simulink subsystem "CiEngineCore"  (R2024a)
settings: Solver=VariableStepAuto  StartTime=0.0  StopTime=10.0  RelTol=1e-3
undefined symbols (not defined in the file): EnvCpAir, EnvRair, PlntEngCEng, PlntEngCIEgrArea, PlntEngCISinj, PlntEngCpExh, PlntEngDieselLhv, PlntEngRexh, PlntEngTauCool, PlntEngTCoolInit, PlntEngTCoolMax, PlntEngTCoolStart, ThrAngToC
libraries: autolibfundflw x11, autolibboost x3, autolibcoreeng x1, simulink x1
settings Model: ModifiedByFormat=The MathWorks, Inc.  Creator=The MathWorks, Inc.  LastModifiedBy=The MathWorks, Inc.
settings SolverCC: MaxZcPerStep=1
settings DebuggingCC: UnconnectedInputMsg=warning  UnconnectedOutputMsg=warning  UnconnectedLineMsg=warning
settings ModelReferenceCC: EnableRefExpFcnMdlSchedulingChecks=on
settings RTWCC: GPUComputeCapability=3.5  DLArmComputeVersion=19.05

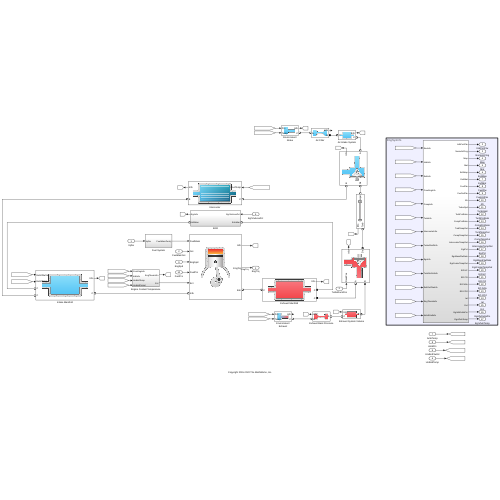
[thumbnail: Simulink's stored preview of the top-level diagram]
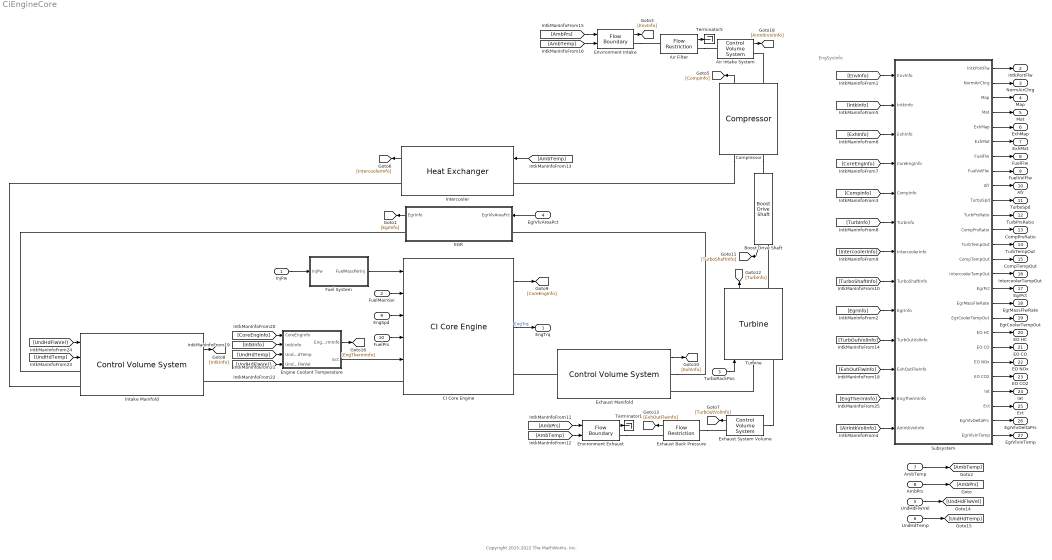
== system CiEngineCore ==
  note: EngSysInfo
  note: Copyright 2015-2022 The MathWorks, Inc.
  InjPw : Inport
  FuelMainSoi : Inport  Port=2
  TurboRackPos : Inport  Port=3
  EgrVlvAreaPct : Inport  Port=4
  UndHdFlwVel : Inport  Port=5
  UndHdTemp : Inport  Port=6
  AmbTemp : Inport  Port=7
  AmbPrs : Inport  Port=8
  EngSpd : Inport  Port=9
  FuelPrs : Inport  Port=10
  Air Filter : autolibfundflw/Flow Restriction  AreaPopup=Constant  ImageTypePopup=Cold  gamma=EnvCpAir/(EnvCpAir-EnvRair)  R=EnvRair  Plim=0.99  Aorf_cnst=PlntEngAFArea  Cd_cnst=1  Cd_ext=1  Dthr=50  ThrCd=[0.001; 0.735]  ThrAngBpts=[0; 90]
  Air Intake System : autolibfundflw/Control Volume System  NumInletPorts=1  NumOutletPorts=1  HeatTransferModelPopup=Constant  ImageTypePopup=Cold  Vch=PlntEngCIAirIntakeVol  Pinit=101325  Tinit=298  R=EnvRair  cp=EnvCpAir  q_he=0  ext_tbl=[40 160 740 2000]  ext_bpts=linspace(0,180,4)  Aext_conv=0.125  m_wall=7  cp_wall=900  Tmass=293.15  Dext_cond=0.004  Aext_cond=0.003  kext=25  Dint_cond=0.004  Aint_cond=0.003  kint=25  int_tbl=[40 160 740 2000]  int_bpts=linspace(0.0020,0.1100,4)  Aint_conv=0.125
  Boost Drive Shaft : autolibboost/Boost Drive Shaft  ShaftConfigPopup=Turbocharger  AddTrqTypePopup=No external torque  J_shaft=PlntEngCITurboInertia  w_0=0.0001  w_min=0.0001  w_max=1e6  eta_mech=1
  CI Core Engine : autolibcoreeng/CI Core Engine  TrqOptionPopup=Torque Structure  NCyl=PlntEngCINCyl  Tstd=EnvAirTemp  Cps=PlntEngCICps  Vd=PlntEngCIVd  Rair=EnvRair  Pstd=EnvAbsPrs  f_nv=PlntEngCINv  f_nv_prs_bpt=PlntEngCINvPrsBpt  f_nv_n_bpt=PlntEngCINvNBpt  f_tq_nf=PlntEngTqNf  f_tq_nf_f_bpt=PlntEngTqNfFBpt  f_tq_nf_n_bpt=PlntEngTqNfNBpt  f_tqs_f_bpt=PlntEngCIGIMepFuelBpt  f_tqs_n_bpt=PlntEngCIGIMepSpdBpt  f_tqs_mainsoi=PlntEngTqsMainSoi  f_tqs_map=PlntEngTqsMap  f_tqs_emap=PlntEngTqsEMap  f_tqs_mat=PlntEngTqsMat  f_tqs_o2pct=PlntEngTqsO2Pct  f_tqs_fuelpress=PlntEngTqsFuelPres  f_tqs_imepg=PlntEngCIGIMepMap  f_tqs_fmep=PlntEngTqsFMep  f_tqs_pmep=PlntEngTqsPMEP  f_tqs_fric_temp_mod=PlntEngTqsFrTmpMod  f_tqs_fric_temp_bpt=PlntEngTqsFrTmpBpt  f_tqs_mainsoi_eff=PlntEngTqsMainSoiEff  f_tqs_mainsoi_delta_bpt=PlntEngTqsMainSoiDeltaBpt  f_tqs_map_eff=PlntEngTqsMapEff  f_tqs_map_ratio_bpt=PlntEngTqsMapRatioBpt  f_tqs_lambda_bpt=PlntEngTqsLambdaBpt  f_tqs_mat_eff=PlntEngTqsMatEff  f_tqs_mat_delta_bpt=PlntEngTqsMatDeltaBpt  f_tqs_o2pct_eff=PlntEngTqsO2PctEff  f_tqs_o2pct_delta_bpt=PlntEngTqsO2PctDeltaBpt  f_tqs_fuelpress_eff=PlntEngTqsFuelPrsEff  f_tqs_fuelpress_delta_bpt=PlntEngTqsFuelPrsDeltaBpt  f_tqs_f_inj_type=PlntEngTqsInjType  f_tqs_imep_post_corr=PlntEngTqsImepPostCorr  f_tqs_f_post_sum_bpt=PlntEngTqsPostSumBpt  f_tqs_soi_post_cent_bpt=PlntEngTqsSoiPostCenBpt  f_tqs_f_burned_soi_limit=PlntEngTqsBurnedSoiLim  f_t_exh=PlntEngCITexh  f_t_exh_f_bpt=PlntEngCITexhFBpt  f_t_exh_n_bpt=PlntEngCITexhNBpt  f_tqs_exht=PlntEngTqsExhT  f_tqs_exht_mainsoi_eff=PlntEngTqsExhTMainSoiEff  f_tqs_exht_map_eff=PlntEngTqsExhTMapEff  f_tqs_exht_mat_eff=PlntEngTqsExhTMatEff  f_tqs_exht_o2pct_eff=PlntEngTqsExhTO2PctEff  f_tqs_exht_fuelpress_eff=PlntEngTqsExhTFuelPrsEff  f_tqs_exht_post_inj_wall_htc=PlntEngTqsExhTPstInjWHtc  CO2EmissionsCheckbox=on  COEmissionsCheckbox=on  NOxEmissionsCheckbox=on  HCEmissionsCheckbox=on  PMEmissionsCheckbox=off  f_CO2_frac=PlntEngCICorefCO2  f_CO_frac=PlntEngCICorefCO  f_HC_frac=PlntEngCICorefHC  f_NOx_frac=PlntEngCICorefNOx  f_PM_frac=[0 0 0 0 0 0 0 0 0 0 0 0 0 0 0;0 0 0 0 0 0 0 0 0 0 0 0 0 0 0;0 0 0 0 0 0 0 0 0 0 0 0 0 0 0;0 0 0 0 0 0 0 0 0 0 0 0 0 0 0;0 0 0 0 0 0 0 0 0 0 0 0 0 0 0;0 0 0 0 0 0 0 0 0 0 0 0 0 0 0;0 0 0 0 0 0 0 0 0 0 0 0 0 0 0;0 0 0 0 0 0 0 0 0 0 0 0 0 0 0;0 0 0 0 0 0 0 0 0 0 0 0 0 0 0;0 0 0 0 0 0 0 0 0 0 0 0 0 0 0;0 0 0 0 0 0 0 0 0 0 0 0 0 0 0;0 0 0 0 0 0 0 0 0 0 0 0 0 0 0;0 0 0 0 0 0 0 0 0 0 0 0 0 0 0;0 0 0 0 0 0 0 0 0 0 0 0 0 0 0;0 0 0 0 0 0 0 0 0 0 0 0 0 0 0;0 0 0 0 0 0 0 0 0 0 0 0 0 0 0]  f_exhfrac_n_bpt=PlntEngCIExhFracNBpt  f_exhfrac_trq_bpt=PlntEngCIExhFracTqBpt  cp_exh=PlntEngCpExh  afr_stoich=PlntEngAfrStoich  fuel_lhv=PlntEngDieselLhv  fuel_sg=0.832
  Compressor : autolibboost/Compressor  mdot_corr_tbl=PlntEngCICompMassFlwRate  eta_comp_tbl=PlntEngCICompEff  w_corr_bpts1=PlntEngCICompSpdBreakPoints  Pr_bpts2=PlntEngCmpPrBpt  T_ref=PlntEngCmpRefT  P_ref=PlntEngCmpRefP  R=EnvRair  cp=EnvCpAir  CalCmprsData={'', '', 'MassFlwRate', 'Eff'}
  EGR : Subsystem
  Engine Coolant Temperature : Subsystem
  Environment Exhaust : autolibfundflw/Flow Boundary  PrsTempSrcPopup=External input  ImageTypePopup=Hot  Pcnst=101325  Tcnst=298.15  cp=EnvCpAir
  Environment Intake : autolibfundflw/Flow Boundary  PrsTempSrcPopup=External input  ImageTypePopup=Cold  Pcnst=101325  Tcnst=298.15  cp=EnvCpAir
  Exhaust Back Pressure : autolibfundflw/Flow Restriction  AreaPopup=Constant  ImageTypePopup=Hot  gamma=PlntEngCpExh/(PlntEngCpExh-PlntEngRexh)  R=PlntEngRexh  Plim=0.99  Aorf_cnst=PlntEngCIExhSysArea  Cd_cnst=1  Cd_ext=1  Dthr=50  ThrCd=[0.001; 0.735]  ThrAngBpts=[0; 90]
  Exhaust Manifold : autolibfundflw/Control Volume System  NumInletPorts=1  NumOutletPorts=2  HeatTransferModelPopup=Constant  ImageTypePopup=Hot  Vch=PlntEngCIVexh  Pinit=101325  Tinit=298  R=PlntEngRexh  cp=PlntEngCpExh  q_he=0  ext_tbl=[40 160 740 2000]  ext_bpts=linspace(0,180,4)  Aext_conv=0.125  m_wall=7  cp_wall=900  Tmass=293.15  Dext_cond=0.004  Aext_cond=0.003  kext=25  Dint_cond=0.004  Aint_cond=0.003  kint=25  int_tbl=[40 160 740 2000]  int_bpts=linspace(0.0020,0.1100,4)  Aint_conv=0.125
  Exhaust System Volume : autolibfundflw/Control Volume System  NumInletPorts=1  NumOutletPorts=1  HeatTransferModelPopup=Constant  ImageTypePopup=Hot  Vch=PlntEngCIExhSysVol  Pinit=101325  Tinit=298  R=PlntEngRexh  cp=PlntEngCpExh  q_he=0  ext_tbl=[40 160 740 2000]  ext_bpts=linspace(0,180,4)  Aext_conv=0.125  m_wall=7  cp_wall=900  Tmass=293.15  Dext_cond=0.004  Aext_cond=0.003  kext=25  Dint_cond=0.004  Aint_cond=0.003  kint=25  int_tbl=[40 160 740 2000]  int_bpts=linspace(0.0020,0.1100,4)  Aint_conv=0.125
  Fuel System : Subsystem
  Intake Manifold : autolibfundflw/Control Volume System  NumInletPorts=2  NumOutletPorts=1  HeatTransferModelPopup=External wall convection  ImageTypePopup=Cold  Vch=PlntEngCIVint  Pinit=101325  Tinit=298  R=EnvRair  cp=EnvCpAir  q_he=0  ext_tbl=[40 160 740 2000]  ext_bpts=linspace(0,180,4)  Aext_conv=0.125  m_wall=7  cp_wall=900  Tmass=293.15  Dext_cond=0.004  Aext_cond=0.003  kext=25  Dint_cond=0.004  Aint_cond=0.003  kint=25  int_tbl=[40 160 740 2000]  int_bpts=linspace(0.0020,0.1100,4)  Aint_conv=0.125
  Intercooler : autolibfundflw/Heat Exchanger  EffctModelPopup=Constant  CoolTempInputPopup=External input  ImageTypePopup=Intercooler  ep_cnst=PlntEngCIIcEffectiveness  T_cool_cnst=PlntEngCoolTemp  cp=EnvCpAir
  Subsystem : Subsystem
  Terminator1 : Terminator
  Terminator5 : Terminator
  Turbine : autolibboost/Turbine  TurbTypePopup=Variable geometry  WgIncludeCheckbox=off  mdot_corrfx_tbl=TurbMassFlwRate  mdot_corrvr_tbl=PlntEngCITurbMassFlwRate  eta_turbfx_tbl=TurbEff  eta_turbvr_tbl=PlntEngCITurbEff  w_corrfx_bpts1=TurbSpdBreakPoints  w_corrvr_bpts2=PlntEngCITurbSpdBreakPoints  Pr_fx_bpts2=TurbPrsRatioBreakPoints  Pr_vr_bpts2=PlntEngCITurbPrsRatioBreakPoints  L_rack_bpts3=PlntEngCITurbRackBreakPoints  T_ref=PlntEngTrbRefT  P_ref=PlntEngTrbRefP  mdot_thresh=1e-6  A_wgopen=WgArea  Plim_wg=.99  R=PlntEngRexh  cp=PlntEngCpExh  CalFixedMapsData={'', '', 'FixedTurbine'}  CalVgtMapsData={'', '', 'Vgt-Point-by-Point'}
  EngTrq : Outport  VectorParamsAs1DForOutWhenUnconnected=off
  IntkPortFlw : Outport  Port=2  VectorParamsAs1DForOutWhenUnconnected=off
  NormAirChrg : Outport  Port=3  VectorParamsAs1DForOutWhenUnconnected=off
  Map : Outport  Port=4  VectorParamsAs1DForOutWhenUnconnected=off
  Mat : Outport  Port=5  VectorParamsAs1DForOutWhenUnconnected=off
  ExhMap : Outport  Port=6  VectorParamsAs1DForOutWhenUnconnected=off
  ExhMat : Outport  Port=7  VectorParamsAs1DForOutWhenUnconnected=off
  FuelFlw : Outport  Port=8  VectorParamsAs1DForOutWhenUnconnected=off
  FuelVolFlw : Outport  Port=9  VectorParamsAs1DForOutWhenUnconnected=off
  Afr : Outport  Port=10  VectorParamsAs1DForOutWhenUnconnected=off
  TurboSpd : Outport  Port=11  VectorParamsAs1DForOutWhenUnconnected=off
  TurbPrsRatio : Outport  Port=12  VectorParamsAs1DForOutWhenUnconnected=off
  CompPrsRatio : Outport  Port=13  VectorParamsAs1DForOutWhenUnconnected=off
  TurbTempOut : Outport  Port=14  VectorParamsAs1DForOutWhenUnconnected=off
  CompTempOut : Outport  Port=15  VectorParamsAs1DForOutWhenUnconnected=off
  IntercoolerTempOut : Outport  Port=16  VectorParamsAs1DForOutWhenUnconnected=off
  EgrPct : Outport  Port=17  VectorParamsAs1DForOutWhenUnconnected=off
  EgrMassFlwRate : Outport  Port=18  VectorParamsAs1DForOutWhenUnconnected=off
  EgrCoolerTempOut : Outport  Port=19  VectorParamsAs1DForOutWhenUnconnected=off
  EO HC : Outport  Port=20  VectorParamsAs1DForOutWhenUnconnected=off
  EO CO : Outport  Port=21  VectorParamsAs1DForOutWhenUnconnected=off
  EO NOx : Outport  Port=22  VectorParamsAs1DForOutWhenUnconnected=off
  EO CO2 : Outport  Port=23  VectorParamsAs1DForOutWhenUnconnected=off
  Iat : Outport  Port=24  VectorParamsAs1DForOutWhenUnconnected=off
  Ect : Outport  Port=25  VectorParamsAs1DForOutWhenUnconnected=off
  EgrVlvDeltaPrs : Outport  Port=26  VectorParamsAs1DForOutWhenUnconnected=off
  EgrVlvInTemp : Outport  Port=27  VectorParamsAs1DForOutWhenUnconnected=off
  wires:
  Subsystem/16(EgrPct) -> EgrPct/1
  Environment Exhaust/1 -> Terminator1/1
  InjPw/1 -> Fuel System/1(InjPw)
  TurboRackPos/1 -> Turbine/1
  Engine Coolant Temperature/2(Ect) -> CI Core Engine/5
  Engine Coolant Temperature/1(EngThermInfo) -> [EngThermInfo]
  UndHdTemp/1 -> [UndHdTemp]
  [UndHdFlwVel] -> Intake Manifold/1
  [IntkInfo] -> Engine Coolant Temperature/2(IntkInfo)
  Subsystem/13(TurbTempOut) -> TurbTempOut/1
  Turbine/1 -> [TurbInfo]
  UndHdFlwVel/1 -> [UndHdFlwVel]
  Subsystem/19(EO HC) -> EO HC/1
  [CoreEngInfo] -> Engine Coolant Temperature/1(CoreEngInfo)
  Subsystem/18(EgrCoolerTempOut) -> EgrCoolerTempOut/1
  Subsystem/24(Ect) -> Ect/1
  [TurboShaftInfo] -> Subsystem/8(TurboShaftInfo)
  Subsystem/6(ExhMat) -> ExhMat/1
  Subsystem/4(Mat) -> Mat/1
  [UndHdTemp] -> Engine Coolant Temperature/3(UndHdTemp)
  Fuel System/1(FuelMassPerInj) -> CI Core Engine/1
  [UndHdFlwVel] -> Engine Coolant Temperature/4(UndHdFlwVel)
  [EgrInfo] -> Subsystem/9(EgrInfo)
  [ExhOutFlwInfo] -> Subsystem/11(ExhOutFlwInfo)
  Subsystem/20(EO CO) -> EO CO/1
  [AmbTemp] -> Environment Intake/2
  Subsystem/11(TurbPrsRatio) -> TurbPrsRatio/1
  FuelMainSoi/1 -> CI Core Engine/2
  [TurbOutVolInfo] -> Subsystem/10(TurbOutVolInfo)
  Subsystem/15(IntercoolerTempOut) -> IntercoolerTempOut/1
  Subsystem/17(EgrMassFlwRate) -> EgrMassFlwRate/1
  Subsystem/2(NormAirChrg) -> NormAirChrg/1
  [CoreEngInfo] -> Subsystem/4(CoreEngInfo)
  [AmbPrs] -> Environment Intake/1
  Subsystem/5(ExhMap) -> ExhMap/1
  Subsystem/9(Afr) -> Afr/1
  AmbTemp/1 -> [AmbTemp]
  Environment Intake/1 -> [EnvInfo]
  [TurbInfo] -> Subsystem/6(TurbInfo)
  Subsystem/1(IntkPortFlw) -> IntkPortFlw/1
  CI Core Engine/1 -> [CoreEngInfo]
  [ExhInfo] -> Subsystem/3(ExhInfo)
  [EnvInfo] -> Subsystem/1(EnvInfo)
  [IntkInfo] -> Subsystem/2(IntkInfo)
  [AmbPrs] -> Environment Exhaust/1
  Exhaust Manifold/1 -> [ExhInfo]
  AmbPrs/1 -> [AmbPrs]
  [CompInfo] -> Subsystem/5(CompInfo)
  Subsystem/21(EO NOx) -> EO NOx/1
  Subsystem/3(Map) -> Map/1
  [AmbTemp] -> Intercooler/1
  EgrVlvAreaPct/1 -> EGR/1(EgrVlvAreaPct)
  EngSpd/1 -> CI Core Engine/3
  Compressor/1 -> [CompInfo]
  Air Filter/1 -> Terminator5/1
  Exhaust Back Pressure/1 -> [ExhOutFlwInfo]
  [EngThermInfo] -> Subsystem/12(EngThermInfo)
  Air Intake System/1 -> [AirIntkVolInfo]
  Intake Manifold/1 -> [IntkInfo]
  Subsystem/8(FuelVolFlw) -> FuelVolFlw/1
  Exhaust System Volume/1 -> [TurbOutVolInfo]
  Subsystem/14(CompTempOut) -> CompTempOut/1
  Subsystem/22(EO CO2) -> EO CO2/1
  EGR/1(EgrInfo) -> [EgrInfo]
  [AmbTemp] -> Environment Exhaust/2
  Subsystem/10(TurboSpd) -> TurboSpd/1
  FuelPrs/1 -> CI Core Engine/4
  Subsystem/12(CompPrsRatio) -> CompPrsRatio/1
  Subsystem/23(Iat) -> Iat/1
  CI Core Engine/2 -> EngTrq/1  "EngTrq"
  [IntercoolerInfo] -> Subsystem/7(IntercoolerInfo)
  [UndHdTemp] -> Intake Manifold/2
  [AirIntkVolInfo] -> Subsystem/13(AirIntkVolInfo)
  Subsystem/25(EgrVlvDeltaPrs) -> EgrVlvDeltaPrs/1
  Intercooler/1 -> [IntercoolerInfo]
  Subsystem/7(FuelFlw) -> FuelFlw/1
  Subsystem/26(EgrVlvInTemp) -> EgrVlvInTemp/1
  Boost Drive Shaft/1 -> [TurboShaftInfo]
  connections:
  Exhaust System Volume/LConn1 -- Turbine/LConn2
  Turbine/LConn1 -- Exhaust Manifold/RConn2
  Exhaust Manifold/LConn1 -- CI Core Engine/RConn1
  Exhaust Back Pressure/LConn1 -- Exhaust System Volume/RConn1
  Intake Manifold/LConn1 -- EGR/RConn1
  Environment Intake/RConn1 -- Air Filter/LConn1
  Compressor/LConn1 -- Intercooler/LConn1
  Exhaust Manifold/RConn1 -- EGR/LConn1
  Intercooler/RConn1 -- Intake Manifold/LConn2
  Compressor/RConn1 -- Air Intake System/RConn1
  Environment Exhaust/RConn1 -- Exhaust Back Pressure/RConn1
  CI Core Engine/LConn1 -- Intake Manifold/RConn1
  Compressor/LConn2 -- Boost Drive Shaft/LConn1
  Air Filter/RConn1 -- Air Intake System/LConn1
  Turbine/RConn1 -- Boost Drive Shaft/RConn1

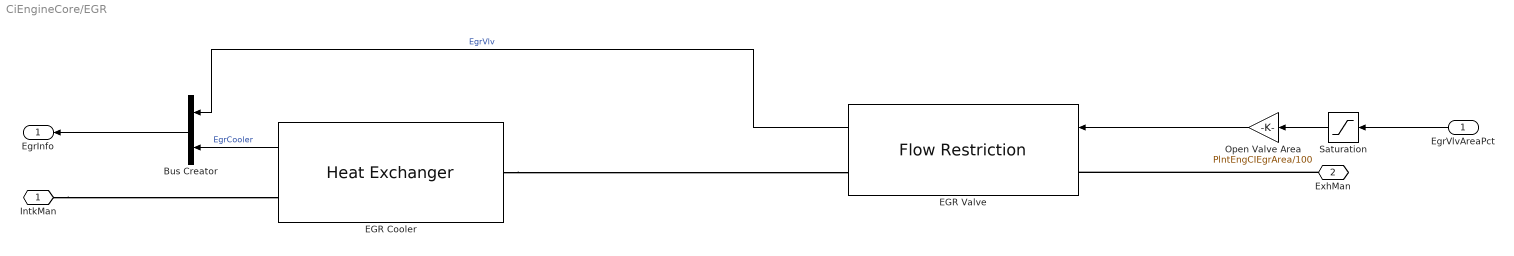
== system CiEngineCore/EGR ==
  EgrVlvAreaPct : Inport
  Bus Creator : BusCreator  Inputs=2
  EGR Cooler : autolibfundflw/Heat Exchanger  EffctModelPopup=Constant  CoolTempInputPopup=Constant  ImageTypePopup=EGR cooler hot to cold  ep_cnst=PlntEngEgrEff  T_cool_cnst=PlntEngREgrCoolT  cp=PlntEngCpExh
  EGR Valve : autolibfundflw/Flow Restriction  AreaPopup=External input  ImageTypePopup=Hot  gamma=PlntEngCpExh / (PlntEngCpExh - PlntEngRexh)  R=EnvRair  Plim=0.99  Aorf_cnst=.1  Cd_cnst=1  Cd_ext=1  Dthr=ThrDiam  ThrCd=ThrAngToC(:,2)  ThrAngBpts=ThrAngToC(:,1)
  Open Valve Area : Gain  Gain=PlntEngCIEgrArea/100
  Saturation : Saturate  UpperLimit=100  LowerLimit=0
  IntkMan : PMIOPort  Side=Right
  ExhMan : PMIOPort  Port=2  Side=Left
  EgrInfo : Outport  VectorParamsAs1DForOutWhenUnconnected=off
  wires:
  EgrVlvAreaPct/1 -> Saturation/1
  Open Valve Area/1 -> EGR Valve/1
  Saturation/1 -> Open Valve Area/1
  Bus Creator/1 -> EgrInfo/1
  EGR Cooler/1 -> Bus Creator/2  "EgrCooler"
  EGR Valve/1 -> Bus Creator/1  "EgrVlv"
  connections:
  EGR Cooler/LConn1 -- EGR Valve/RConn1
  IntkMan/RConn1 -- EGR Cooler/RConn1
  ExhMan/RConn1 -- EGR Valve/LConn1

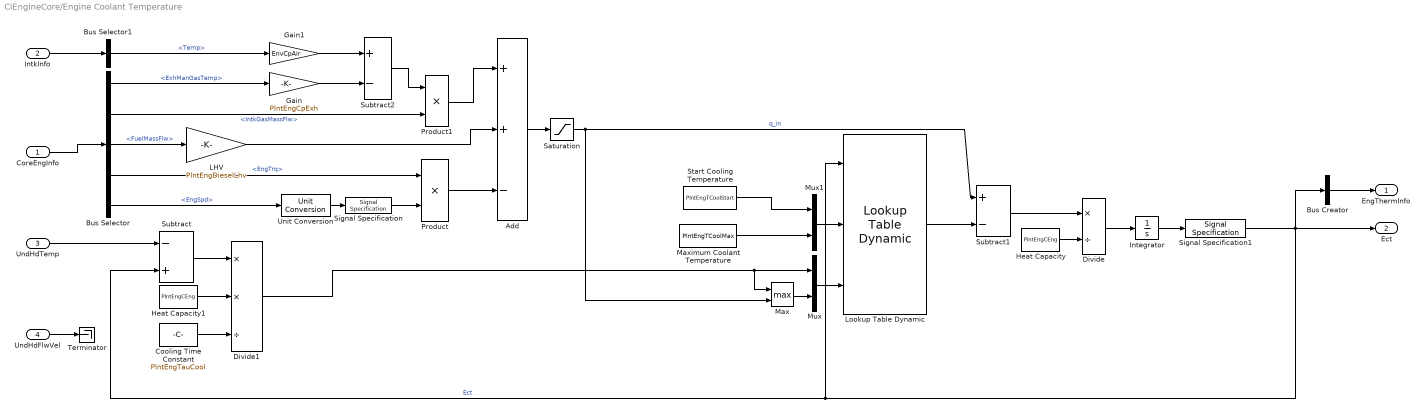
== system CiEngineCore/Engine Coolant Temperature ==
  CoreEngInfo : Inport
  IntkInfo : Inport  Port=2
  UndHdTemp : Inport  Port=3
  UndHdFlwVel : Inport  Port=4
  Add : Sum  Inputs=++-
  Bus Creator : BusCreator  Inputs=1
  Bus Selector : BusSelector  OutputSignals=ExhManGasTemp,IntkGasMassFlw,FuelMassFlw,EngTrq,EngSpd
  Bus Selector1 : BusSelector  OutputSignals=Vol.Temp
  Cooling Time Constant : Constant  Value=PlntEngTauCool
  Divide : Product  Inputs=*/
  Divide1 : Product  Inputs=**/
  Gain : Gain  Gain=PlntEngCpExh
  Gain1 : Gain  Gain=EnvCpAir
  Heat Capacity : Constant  Value=PlntEngCEng
  Heat Capacity1 : Constant  Value=PlntEngCEng
  Integrator : Integrator  InitialCondition=PlntEngTCoolInit  LimitOutput=on  UpperSaturationLimit=PlntEngTCoolMax  LowerSaturationLimit=0  ZeroCross=off
  LHV : Gain  Gain=PlntEngDieselLhv
  Lookup Table Dynamic : simulink/Lookup Tables/Lookup Table Dynamic  LookUpMeth=Interpolation-Use End Values  OutDataType=fixdt('double')  OutScaling=[]  OutputDataTypeScalingMode=Specify via dialog  OutDataTypeStr=double  DoSatur=off
  Max : MinMax  Function=max  Inputs=2  ZeroCross=off
  Maximum Coolant Temperature : Constant  Value=PlntEngTCoolMax
  Mux : Mux  Inputs=2
  Mux1 : Mux  Inputs=2
  Product : Product
  Product1 : Product
  Saturation : Saturate  UpperLimit=Inf  LowerLimit=0
  Signal Specification : SignalSpecification  Unit=rad/s
  Signal Specification1 : SignalSpecification  Unit=K
  Start Cooling Temperature : Constant  Value=PlntEngTCoolStart
  Subtract : Sum  Inputs=-+
  Subtract1 : Sum  Inputs=+-
  Subtract2 : Sum  Inputs=+-
  Terminator : Terminator
  Unit Conversion : UnitConversion
  EngThermInfo : Outport  Unit=K  VectorParamsAs1DForOutWhenUnconnected=off
  Ect : Outport  Port=2  Unit=K  VectorParamsAs1DForOutWhenUnconnected=off
  wires:
  UndHdTemp/1 -> Subtract/1
  Heat Capacity/1 -> Divide/2
  Unit Conversion/1 -> Signal Specification/1
  Maximum Coolant Temperature/1 -> Mux1/2
  Signal Specification1/1 -> Subtract/2, Lookup Table Dynamic/1, Bus Creator/1, Ect/1  "Ect"
  UndHdFlwVel/1 -> Terminator/1
  Gain/1 -> Subtract2/2
  Bus Selector/4 -> Product/1  "<EngTrq>"
  Mux1/1 -> Lookup Table Dynamic/2
  Divide1/1 -> Max/1, Mux/1
  Heat Capacity1/1 -> Divide1/2
  Mux/1 -> Lookup Table Dynamic/3
  Start Cooling Temperature/1 -> Mux1/1
  Subtract/1 -> Divide1/1
  Saturation/1 -> Max/2, Subtract1/1  "q_in"
  Signal Specification/1 -> Product/2
  LHV/1 -> Add/2
  Product/1 -> Add/3
  Bus Selector/5 -> Unit Conversion/1  "<EngSpd>"
  Cooling Time Constant/1 -> Divide1/3
  CoreEngInfo/1 -> Bus Selector/1
  Bus Selector/3 -> LHV/1  "<FuelMassFlw>"
  Bus Selector/1 -> Gain/1  "<ExhManGasTemp>"
  Gain1/1 -> Subtract2/1
  Bus Selector1/1 -> Gain1/1  "<Temp>"
  Divide/1 -> Integrator/1
  Subtract1/1 -> Divide/1
  Lookup Table Dynamic/1 -> Subtract1/2
  Max/1 -> Mux/2
  Bus Creator/1 -> EngThermInfo/1
  IntkInfo/1 -> Bus Selector1/1
  Integrator/1 -> Signal Specification1/1
  Subtract2/1 -> Product1/1
  Bus Selector/2 -> Product1/2  "<IntkGasMassFlw>"
  Product1/1 -> Add/1
  Add/1 -> Saturation/1

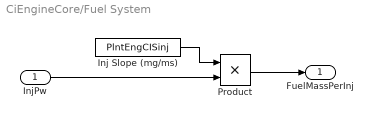
== system CiEngineCore/Fuel System ==
  InjPw : Inport
  Inj Slope (mg/ms) : Constant  Value=PlntEngCISinj
  Product : Product
  FuelMassPerInj : Outport  VectorParamsAs1DForOutWhenUnconnected=off
  wires:
  InjPw/1 -> Product/2
  Inj Slope (mg/ms)/1 -> Product/1
  Product/1 -> FuelMassPerInj/1

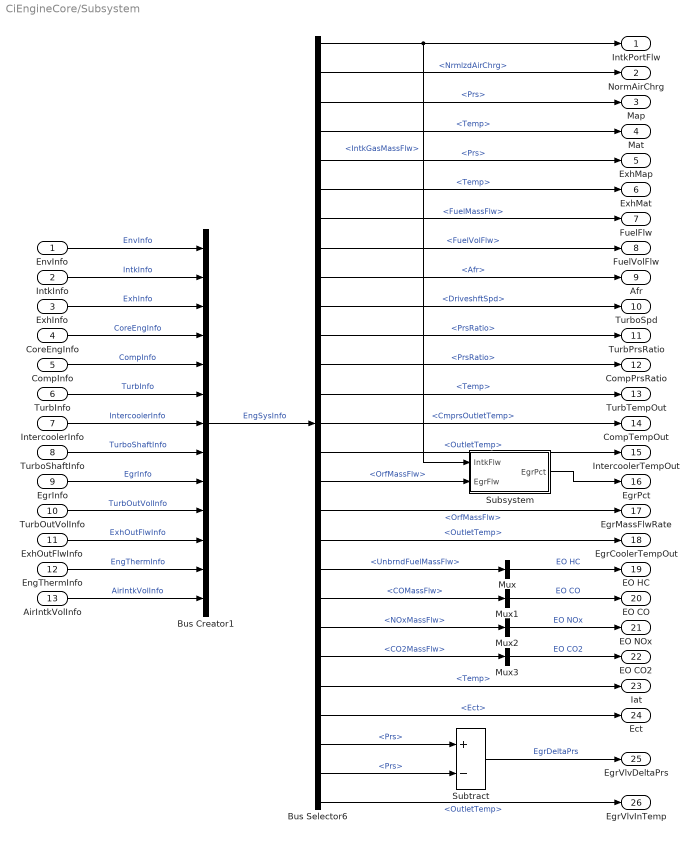
== system CiEngineCore/Subsystem ==
  EnvInfo : Inport
  IntkInfo : Inport  Port=2
  ExhInfo : Inport  Port=3
  CoreEngInfo : Inport  Port=4
  CompInfo : Inport  Port=5
  TurbInfo : Inport  Port=6
  IntercoolerInfo : Inport  Port=7
  TurboShaftInfo : Inport  Port=8
  EgrInfo : Inport  Port=9
  TurbOutVolInfo : Inport  Port=10
  ExhOutFlwInfo : Inport  Port=11
  EngThermInfo : Inport  Port=12
  AirIntkVolInfo : Inport  Port=13
  Bus Creator1 : BusCreator  Inputs=13
  Bus Selector6 : BusSelector  OutputSignals=CoreEngInfo.IntkGasMassFlw,CoreEngInfo.NrmlzdAirChrg,IntkInfo.Vol.Prs,IntkInfo.Vol.Temp,ExhInfo.Vol.Prs,ExhInfo.Vol.Temp,CoreEngInfo.FuelMassFlw,CoreEngInfo.FuelVolFlw,CoreEngInfo.Afr,TurboShaftInfo.DriveshftSpd,TurbInfo.PrsRatio,CompInfo.PrsRatio,TurbOutVolInfo.Vol.Temp,CompInfo.CmprsOutletTemp,IntercoolerInfo.OutletTemp,EgrInfo.EgrVlv.Flw.OrfMassFlw,EgrInfo.EgrVlv.Flw.OrfMassFlw,EgrInfo.EgrCooler.OutletTemp,ExhOutFlwInfo.Flw.Species.UnbrndFuelMassFlw,ExhOutFlwInfo.Flw.Species.COMassFlw,ExhOutFlwInfo.Flw.Species.NOxMassFlw,ExhOutFlwInfo.Flw.Species.CO2MassFlw,AirIntkVolInfo.Vol.Temp,EngThermInfo.Ect,ExhInfo.Vol.Prs,IntkInfo.Vol.Prs,EgrInfo.EgrCooler.OutletTemp
  Mux{,1..3} (4 alike) : Mux  Inputs=1
  Subsystem : Subsystem
  Subtract : Sum  Inputs=+-
  IntkPortFlw : Outport  VectorParamsAs1DForOutWhenUnconnected=off
  NormAirChrg : Outport  Port=2  Unit=1  VectorParamsAs1DForOutWhenUnconnected=off
  Map : Outport  Port=3  VectorParamsAs1DForOutWhenUnconnected=off
  Mat : Outport  Port=4  VectorParamsAs1DForOutWhenUnconnected=off
  ExhMap : Outport  Port=5  VectorParamsAs1DForOutWhenUnconnected=off
  ExhMat : Outport  Port=6  VectorParamsAs1DForOutWhenUnconnected=off
  FuelFlw : Outport  Port=7  VectorParamsAs1DForOutWhenUnconnected=off
  FuelVolFlw : Outport  Port=8  VectorParamsAs1DForOutWhenUnconnected=off
  Afr : Outport  Port=9  Unit=1  VectorParamsAs1DForOutWhenUnconnected=off
  TurboSpd : Outport  Port=10  VectorParamsAs1DForOutWhenUnconnected=off
  TurbPrsRatio : Outport  Port=11  VectorParamsAs1DForOutWhenUnconnected=off
  CompPrsRatio : Outport  Port=12  VectorParamsAs1DForOutWhenUnconnected=off
  TurbTempOut : Outport  Port=13  VectorParamsAs1DForOutWhenUnconnected=off
  CompTempOut : Outport  Port=14  VectorParamsAs1DForOutWhenUnconnected=off
  IntercoolerTempOut : Outport  Port=15  VectorParamsAs1DForOutWhenUnconnected=off
  EgrPct : Outport  Port=16  Unit=%  VectorParamsAs1DForOutWhenUnconnected=off
  EgrMassFlwRate : Outport  Port=17  VectorParamsAs1DForOutWhenUnconnected=off
  EgrCoolerTempOut : Outport  Port=18  VectorParamsAs1DForOutWhenUnconnected=off
  EO HC : Outport  Port=19  VectorParamsAs1DForOutWhenUnconnected=off
  EO CO : Outport  Port=20  VectorParamsAs1DForOutWhenUnconnected=off
  EO NOx : Outport  Port=21  VectorParamsAs1DForOutWhenUnconnected=off
  EO CO2 : Outport  Port=22  VectorParamsAs1DForOutWhenUnconnected=off
  Iat : Outport  Port=23  VectorParamsAs1DForOutWhenUnconnected=off
  Ect : Outport  Port=24  VectorParamsAs1DForOutWhenUnconnected=off
  EgrVlvDeltaPrs : Outport  Port=25  Unit=Pa  VectorParamsAs1DForOutWhenUnconnected=off
  EgrVlvInTemp : Outport  Port=26  Unit=K  VectorParamsAs1DForOutWhenUnconnected=off
  wires:
  TurbOutVolInfo/1 -> Bus Creator1/10  "TurbOutVolInfo"
  EgrInfo/1 -> Bus Creator1/9  "EgrInfo"
  Bus Selector6/15 -> IntercoolerTempOut/1  "<OutletTemp>"
  Bus Selector6/14 -> CompTempOut/1  "<CmprsOutletTemp>"
  Bus Selector6/13 -> TurbTempOut/1  "<Temp>"
  Bus Selector6/12 -> CompPrsRatio/1  "<PrsRatio>"
  Bus Selector6/11 -> TurbPrsRatio/1  "<PrsRatio>"
  Bus Selector6/2 -> NormAirChrg/1  "<NrmlzdAirChrg>"
  Bus Selector6/9 -> Afr/1  "<Afr>"
  Bus Selector6/7 -> FuelFlw/1  "<FuelMassFlw>"
  Bus Selector6/6 -> ExhMat/1  "<Temp>"
  Bus Selector6/5 -> ExhMap/1  "<Prs>"
  Bus Selector6/4 -> Mat/1  "<Temp>"
  Bus Selector6/3 -> Map/1  "<Prs>"
  Bus Selector6/1 -> Subsystem/1(IntkFlw), IntkPortFlw/1  "<IntkGasMassFlw>"
  TurboShaftInfo/1 -> Bus Creator1/8  "TurboShaftInfo"
  TurbInfo/1 -> Bus Creator1/6  "TurbInfo"
  IntercoolerInfo/1 -> Bus Creator1/7  "IntercoolerInfo"
  Bus Creator1/1 -> Bus Selector6/1  "EngSysInfo"
  EnvInfo/1 -> Bus Creator1/1  "EnvInfo"
  CoreEngInfo/1 -> Bus Creator1/4  "CoreEngInfo"
  ExhInfo/1 -> Bus Creator1/3  "ExhInfo"
  IntkInfo/1 -> Bus Creator1/2  "IntkInfo"
  CompInfo/1 -> Bus Creator1/5  "CompInfo"
  Bus Selector6/18 -> EgrCoolerTempOut/1  "<OutletTemp>"
  ExhOutFlwInfo/1 -> Bus Creator1/11  "ExhOutFlwInfo"
  Bus Selector6/19 -> Mux/1  "<UnbrndFuelMassFlw>"
  Bus Selector6/20 -> Mux1/1  "<COMassFlw>"
  Bus Selector6/21 -> Mux2/1  "<NOxMassFlw>"
  Bus Selector6/22 -> Mux3/1  "<CO2MassFlw>"
  Mux/1 -> EO HC/1  "EO HC"
  Mux1/1 -> EO CO/1  "EO CO"
  Mux2/1 -> EO NOx/1  "EO NOx"
  Mux3/1 -> EO CO2/1  "EO CO2"
  Bus Selector6/10 -> TurboSpd/1  "<DriveshftSpd>"
  Bus Selector6/24 -> Ect/1  "<Ect>"
  EngThermInfo/1 -> Bus Creator1/12  "EngThermInfo"
  Bus Selector6/17 -> EgrMassFlwRate/1  "<OrfMassFlw>"
  Subtract/1 -> EgrVlvDeltaPrs/1  "EgrDeltaPrs"
  Bus Selector6/27 -> EgrVlvInTemp/1  "<OutletTemp>"
  Bus Selector6/26 -> Subtract/2  "<Prs>"
  Bus Selector6/25 -> Subtract/1  "<Prs>"
  Subsystem/1(EgrPct) -> EgrPct/1
  Bus Selector6/16 -> Subsystem/2(EgrFlw)  "<OrfMassFlw>"
  AirIntkVolInfo/1 -> Bus Creator1/13  "AirIntkVolInfo"
  Bus Selector6/23 -> Iat/1  "<Temp>"
  Bus Selector6/8 -> FuelVolFlw/1  "<FuelVolFlw>"

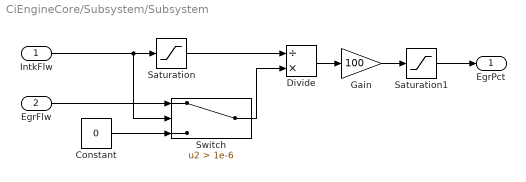
== system CiEngineCore/Subsystem/Subsystem ==
  IntkFlw : Inport
  EgrFlw : Inport  Port=2
  Constant : Constant  Value=0
  Divide : Product  Inputs=/*
  Gain : Gain  Gain=100
  Saturation : Saturate  UpperLimit=1e6  LowerLimit=1e-6  ZeroCross=off
  Saturation1 : Saturate  UpperLimit=100  LowerLimit=0  ZeroCross=off
  Switch : Switch  Criteria=u2 > Threshold  Threshold=1e-6  ZeroCross=off  SaturateOnIntegerOverflow=off  InputSameDT=off
  EgrPct : Outport  VectorParamsAs1DForOutWhenUnconnected=off
  wires:
  Constant/1 -> Switch/3
  Divide/1 -> Gain/1
  Switch/1 -> Divide/2
  Saturation/1 -> Divide/1
  Gain/1 -> Saturation1/1
  EgrFlw/1 -> Switch/1
  IntkFlw/1 -> Switch/2, Saturation/1
  Saturation1/1 -> EgrPct/1
